simulink model "derpage3"  (R2016a)
settings: Solver=FixedStepDiscrete  SolverMode=SingleTasking  StartTime=0.0  StopTime=(12+4)*8-1  RelTol=1e-3
undefined symbols (not defined in the file or in its folder): rcosine
libraries: dspstat3 x1, dspsrcs4 x1, dspsigops x1
settings Model: Creator=coltmt  LastModifiedBy=coltmt
settings DataIOCC: LimitDataPoints=on
settings DebuggingCC: AllowSymbolicDim=off
settings ModelReferenceCC: PropagateSignalLabelsOutOfModel=off
settings GRTTargetCC: GeneratePreprocessorConditionals=Use local settings

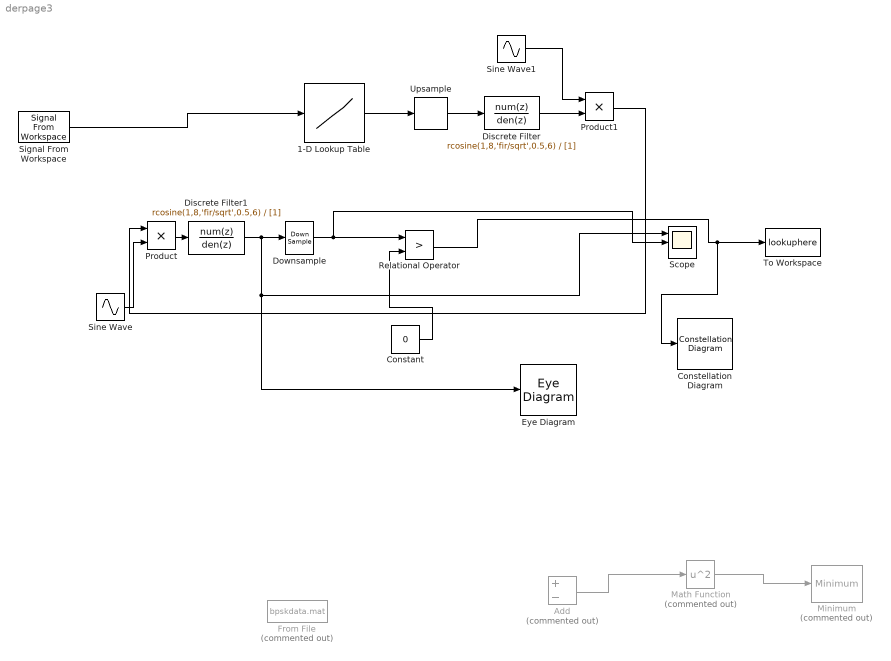
== system derpage3 ==
  1-D Lookup Table : Lookup_n-D  NumberOfTableDimensions=1  BreakpointsForDimension1=[0:1]  Table=[-1 1]  InternalRulePriority=Speed  RndMeth=Simplest  InputSameDT=on
  Add : Sum  Commented=on  Inputs=+-
  Constant : Constant  Value=0
  Constellation Diagram : ConstellationDiagram
  Discrete Filter : DiscreteFilter  Numerator=rcosine(1,8,'fir/sqrt',0.5,6)  Denominator=[1]
  Discrete Filter1 : DiscreteFilter  Numerator=rcosine(1,8,'fir/sqrt',0.5,6)  Denominator=[1]
  Downsample : DownSample  N=8  phase=1  InputProcessing=Inherited (this choice will be removed - see release notes)  RateOptions=Allow multirate processing
  Eye Diagram : EyeDiagram
  From File : FromFile  Commented=on  FileName=bpskdata.mat  OutDataTypeStr=double  SampleTime=1
  Math Function : Math  Commented=on  Operator=square  SaturateOnIntegerOverflow=on
  Minimum : dspstat3/Minimum  Commented=on  fcn=Index  reset=None  InputProcessing=Columns as channels (frame based)  indexBase=Zero  operateOver=Each column  Dimension=1  operation=minimum  roiEnable=off  roiType=Rectangles  roiPortion=Entire ROI  roiOutput=Individual statistics for each ROI  roiFlag=off  roundingMode=Floor  overflowMode=off
  Product : Product
  Product1 : Product
  Relational Operator : RelationalOperator  Operator=>  OutDataTypeStr=boolean
  Scope : Scope  NumInputPorts=3
  Signal From Workspace : dspsrcs4/Signal From Workspace  X=[1 0 0 1]  Ts=1  nsamps=1  OutputAfterFinalValue=Setting to zero  ignoreOrWarnInputAndFrameLengths=off  OutputFrames=off
  Sine Wave : Sin  Amplitude=sqrt(2)  Frequency=2*pi/4  Phase=pi/2  SampleTime=1
  Sine Wave1 : Sin  Amplitude=sqrt(2)  Frequency=2*pi/4  Phase=pi/2  SampleTime=1
  To Workspace : ToWorkspace  VariableName=lookuphere  SampleTime=-1
      settings: Save2DSignal=2-D array (concatenate along first dimension)
  Upsample : dspsigops/Upsample  N=8  phase=0  InputProcessing=Inherited (this choice will be removed - see release notes)  RateOptions=Allow multirate processing  ic=0  mode=Unused parameter value
  wires:
  1-D Lookup Table/1 -> Upsample/1
  Upsample/1 -> Discrete Filter/1
  Discrete Filter1/1 -> Scope/1, Eye Diagram/1, Downsample/1
  Downsample/1 -> Scope/2, Relational Operator/1
  Add/1 -> Math Function/1
  Math Function/1 -> Minimum/1
  Sine Wave/1 -> Product/2
  Product/1 -> Discrete Filter1/1
  Discrete Filter/1 -> Product1/2
  Sine Wave1/1 -> Product1/1
  Relational Operator/1 -> Constellation Diagram/1, To Workspace/1
  Constant/1 -> Relational Operator/2
  Signal From Workspace/1 -> 1-D Lookup Table/1
  Product1/1 -> Product/1
